simulink library "aerolibgravity2"  (R2020a)
settings: Solver=ode45  StartTime=0.0  StopTime=10.0  RelTol=1e-3
PostLoadFcn:
  | load_system('aerolibv1')
  | setsysloc('aerolibv1')
undefined symbols (not defined in the file or in its folder): aeroassertmsg, C, geoidgrid, ghCurrent, GM, latbp, lonbp, minYearCurrent, Newton, nMax10, nMax13, nMaxBetween, nMaxCurrent, R, Raphson, S, svCurrent, tabNMax10, tabNMax13, tabNMaxBetween
libraries: simulink x17, aerolibgravitysys x4
(part 3 of 4)

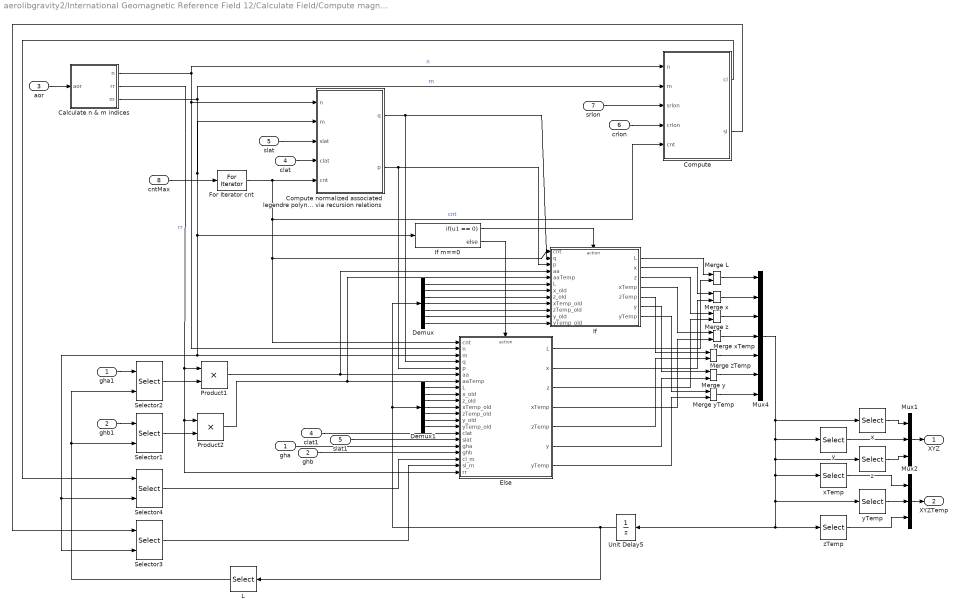
== system aerolibgravity2/International Geomagnetic Reference Field 12/Calculate Field/Compute magnetic vector in spherical coordinates/Compute magnetic vector in spherical coordinates ==
  gha : Inport  PortDimensions=(nMax13+1)*(nMax13+1)-1
  ghb : Inport  Port=2  PortDimensions=(nMax13+1)*(nMax13+1)-1
  aor : Inport  Port=3
  clat : Inport  Port=4
  slat : Inport  Port=5
  crlon : Inport  Port=6
  srlon : Inport  Port=7
  cntMax : Inport  Port=8
  Calculate n & m indices : Subsystem
  "Compute " : Subsystem
  Compute normalized associated legendre polynomials and derivatives via recursion relations : Subsystem
  Demux : Demux  Outputs=7
  Demux1 : Demux  Outputs=7
  Else : Subsystem
  For Iterator cnt : ForIterator  ResetStates=reset  IterationSource=external  IterationLimit=nPG
  If : Subsystem
  If m==0 : If  IfExpression=u1 == 0
  L : Selector  InputPortWidth=7  IndexOptions=Index vector (dialog)  Indices=1  OutputSizes=1
  Merge L : Merge  InitialOutput=0
  Merge x : Merge  InitialOutput=0
  Merge xTemp : Merge  InitialOutput=0
  Merge y : Merge  InitialOutput=0
  Merge yTemp : Merge  InitialOutput=0
  Merge z : Merge  InitialOutput=0
  Merge zTemp : Merge  InitialOutput=0
  Mux1 : Mux  Inputs=3
  Mux2 : Mux  Inputs=3
  Mux4 : Mux  Inputs=7
  Product1 : Product  SaturateOnIntegerOverflow=on  OutDataTypeStr=Inherit: Same as first input
  Product2 : Product  SaturateOnIntegerOverflow=on  OutDataTypeStr=Inherit: Same as first input
  Selector1 : Selector  InputPortWidth=(nMax13+1)*(nMax13+1)-1  IndexOptions=Index vector (port)  Indices=[1 3]  OutputSizes=1
  Selector2 : Selector  InputPortWidth=(nMax13+1)*(nMax13+1)-1  IndexOptions=Index vector (port)  Indices=[1 3]  OutputSizes=1
  Selector3 : Selector  IndexMode=Zero-based  InputPortWidth=nMax13+1  IndexOptions=Index vector (port)  Indices=[1 3]  OutputSizes=1
  Selector4 : Selector  IndexMode=Zero-based  InputPortWidth=nMax13+1  IndexOptions=Index vector (port)  Indices=[1 3]  OutputSizes=1
  Unit Delay5 : UnitDelay  InitialCondition=[1 0 0 0 0 0 0]  SampleTime=-1  HasFrameUpgradeWarning=on
  clat1 : InportShadow  Port=4
  gha1 : InportShadow  PortDimensions=(nMax13+1)*(nMax13+1)-1
  ghb1 : InportShadow  Port=2  PortDimensions=(nMax13+1)*(nMax13+1)-1
  slat1 : InportShadow  Port=5
  x : Selector  InputPortWidth=7  IndexOptions=Index vector (dialog)  Indices=2  OutputSizes=1
  xTemp : Selector  InputPortWidth=7  IndexOptions=Index vector (dialog)  Indices=4  OutputSizes=1
  y : Selector  InputPortWidth=7  IndexOptions=Index vector (dialog)  Indices=6  OutputSizes=1
  yTemp : Selector  InputPortWidth=7  IndexOptions=Index vector (dialog)  Indices=7  OutputSizes=1
  z : Selector  InputPortWidth=7  IndexOptions=Index vector (dialog)  Indices=3  OutputSizes=1
  zTemp : Selector  InputPortWidth=7  IndexOptions=Index vector (dialog)  Indices=5  OutputSizes=1
  XYZ : Outport  InitialOutput=[0 0 0]  VectorParamsAs1DForOutWhenUnconnected=off
  XYZTemp : Outport  Port=2  InitialOutput=[0 0 0]  VectorParamsAs1DForOutWhenUnconnected=off
  wires:
  yTemp/1 -> Mux2/2
  y/1 -> Mux1/2
  Demux1/7 -> Else/14(yTemp_old)
  Demux1/6 -> Else/13(y_old)
  Demux/7 -> If/12(yTemp_old)
  Demux/6 -> If/11(y_old)
  If/7(yTemp) -> Merge yTemp/1
  If/6(y) -> Merge y/1
  Else/7(yTemp) -> Merge yTemp/2
  cntMax/1 -> For Iterator cnt/1
  clat/1 -> Compute normalized associated legendre polynomials and derivatives via recursion relations/4(clat)
  slat/1 -> Compute normalized associated legendre polynomials and derivatives via recursion relations/3(slat)
  gha/1 -> Else/17(gha)
  ghb/1 -> Else/18(ghb)
  Mux2/1 -> XYZTemp/1
  Mux1/1 -> XYZ/1
  For Iterator cnt/1 -> Compute normalized associated legendre polynomials and derivatives via recursion relations/5(cnt), Else/1(cnt), If/1(cnt), "Compute "/5(cnt)  "cnt"
  If m==0/1 -> If/Action
  If m==0/2 -> Else/Action
  If/1("L ") -> Merge L/1
  If/2(x) -> Merge x/1
  If/3(z) -> Merge z/1
  If/4(xTemp) -> Merge xTemp/1
  If/5(zTemp) -> Merge zTemp/1
  Else/1("L ") -> Merge L/2
  Else/2(x) -> Merge x/2
  Else/3(z) -> Merge z/2
  Else/4(xTemp) -> Merge xTemp/2
  Else/5(zTemp) -> Merge zTemp/2
  Mux4/1 -> y/1, yTemp/1, Unit Delay5/1, zTemp/1, xTemp/1, z/1, x/1
  Else/6(y) -> Merge y/2
  Unit Delay5/1 -> Demux1/1, Demux/1, L/1
  Demux/1 -> If/6(L)
  Demux/3 -> If/8(z_old)
  Demux/2 -> If/7(x_old)
  Demux/4 -> If/9(xTemp_old)
  Demux/5 -> If/10(zTemp_old)
  Demux1/1 -> Else/8(L)
  Demux1/5 -> Else/12(zTemp_old)
  Demux1/4 -> Else/11(xTemp_old)
  Demux1/3 -> Else/10(z_old)
  Demux1/2 -> Else/9(x_old)
  xTemp/1 -> Mux2/1
  zTemp/1 -> Mux2/3
  x/1 -> Mux1/1
  z/1 -> Mux1/3
  Compute normalized associated legendre polynomials and derivatives via recursion relations/1(q) -> If/2(q), Else/4(q)
  Compute normalized associated legendre polynomials and derivatives via recursion relations/2(p) -> If/3(p), Else/5(p)
  Calculate n & m indices/2(rr) -> Product1/1, Else/21(rr), Product2/1  "rr"
  clat1/1 -> Else/15(clat)
  slat1/1 -> Else/16(slat)
  gha1/1 -> Selector2/1
  ghb1/1 -> Selector1/1
  L/1 -> Selector2/2, Selector1/2
  Selector2/1 -> Product1/2
  Product1/1 -> Else/6(aa), If/4(aa)
  Selector1/1 -> Product2/2
  Product2/1 -> Else/7(aaTemp), If/5(aaTemp)
  srlon/1 -> "Compute "/3(srlon)
  crlon/1 -> "Compute "/4(crlon)
  "Compute "/1(cl) -> Selector4/1
  Selector4/1 -> Else/19(cl_m)
  Selector3/1 -> Else/20(sl_m)
  "Compute "/2(sl) -> Selector3/1
  Calculate n & m indices/1(n) -> Else/2(n), Compute normalized associated legendre polynomials and derivatives via recursion relations/1(n), "Compute "/1(n)  "n"
  Calculate n & m indices/3(m) -> Compute normalized associated legendre polynomials and derivatives via recursion relations/2(m), Else/3(m), Selector4/2, Selector3/2, If m==0/1, "Compute "/2(m)  "m"
  aor/1 -> Calculate n & m indices/1(aor)
  Merge L/1 -> Mux4/1
  Merge x/1 -> Mux4/2
  Merge z/1 -> Mux4/3
  Merge y/1 -> Mux4/6
  Merge yTemp/1 -> Mux4/7
  Merge zTemp/1 -> Mux4/5
  Merge xTemp/1 -> Mux4/4

== system aerolibgravity2/International Geomagnetic Reference Field 12/Calculate Field/Convert from geodetic to spherical coordinates/calculate cd ==
  alt : Inport
  r : Inport  Port=2
  d : Inport  Port=3
  Product11 : Product  Inputs=*/  OutDataTypeStr=Inherit: Inherit via back propagation  SaturateOnIntegerOverflow=on
  Sum8 : Sum  Inputs=|++  OutDataTypeStr=Inherit: Inherit via back propagation  SaturateOnIntegerOverflow=on
  cd : Outport  VectorParamsAs1DForOutWhenUnconnected=off
  wires:
  Product11/1 -> cd/1
  d/1 -> Sum8/2
  alt/1 -> Sum8/1
  r/1 -> Product11/2
  Sum8/1 -> Product11/1

== system aerolibgravity2/International Geomagnetic Reference Field 12/Calculate Field/Convert from geodetic to spherical coordinates/calculate clat & slat ==
  sd : Inport
  srlat : Inport  Port=2
  crlat : Inport  Port=3
  cd : Inport  Port=4
  Product{1..4} (4 alike) : Product  OutDataTypeStr=Inherit: Inherit via back propagation  SaturateOnIntegerOverflow=on
  Sum1 : Sum  Inputs=|+-  OutDataTypeStr=Inherit: Inherit via back propagation  SaturateOnIntegerOverflow=on
  Sum2 : Sum  Inputs=|++  OutDataTypeStr=Inherit: Inherit via back propagation  SaturateOnIntegerOverflow=on
  "cd " : InportShadow  Port=4
  "crlat " : InportShadow  Port=3
  "sd " : InportShadow
  "srlat " : InportShadow  Port=2
  clat : Outport  VectorParamsAs1DForOutWhenUnconnected=off
  slat : Outport  Port=2  VectorParamsAs1DForOutWhenUnconnected=off
  wires:
  srlat/1 -> Product1/1
  cd/1 -> Product1/2
  sd/1 -> Product2/2
  crlat/1 -> Product2/1
  Product1/1 -> Sum1/1
  Product2/1 -> Sum1/2
  Sum1/1 -> slat/1
  "crlat "/1 -> Product3/1
  "cd "/1 -> Product3/2
  "srlat "/1 -> Product4/1
  "sd "/1 -> Product4/2
  Product4/1 -> Sum2/1
  Product3/1 -> Sum2/2
  Sum2/1 -> clat/1

== system aerolibgravity2/International Geomagnetic Reference Field 12/Calculate Field/Convert from geodetic to spherical coordinates/calculate d ==
  a2 : Inport
  b2 : Inport  Port=2
  srlat2 : Inport  Port=3
  crlat2 : Inport  Port=4
  Product10 : Product  OutDataTypeStr=Inherit: Inherit via back propagation  SaturateOnIntegerOverflow=on
  Product9 : Product  OutDataTypeStr=Inherit: Inherit via back propagation  SaturateOnIntegerOverflow=on
  Sum7 : Sum  Inputs=++|  OutDataTypeStr=Inherit: Inherit via back propagation  SaturateOnIntegerOverflow=on
  sqrt : Sqrt  OutDataTypeStr=Inherit: Inherit via back propagation  AlgorithmType=Newton-Raphson  SaturateOnIntegerOverflow=on
  c2 : Outport  VectorParamsAs1DForOutWhenUnconnected=off
  d : Outport  Port=2  VectorParamsAs1DForOutWhenUnconnected=off
  wires:
  sqrt/1 -> d/1  "d"
  srlat2/1 -> Product10/2
  b2/1 -> Product10/1
  a2/1 -> Product9/2
  crlat2/1 -> Product9/1
  Product10/1 -> Sum7/2
  Product9/1 -> Sum7/1
  Sum7/1 -> sqrt/1, c2/1

== system aerolibgravity2/International Geomagnetic Reference Field 12/Calculate Field/Convert from geodetic to spherical coordinates/calculate r2 ==
  alt : Inport
  a2 : Inport  Port=2
  b2 : Inport  Port=3
  srlat2 : Inport  Port=4
  crlat2 : Inport  Port=5
  c2 : Inport  Port=6
  d : Inport  Port=7
  Gain : Gain  Gain=2  OutDataTypeStr=Inherit: Inherit via back propagation  SaturateOnIntegerOverflow=on
  Product1 : Product  OutDataTypeStr=Inherit: Inherit via back propagation  SaturateOnIntegerOverflow=on
  Product2 : Product  OutDataTypeStr=Inherit: Inherit via back propagation  SaturateOnIntegerOverflow=on
  Product7 : Product  Inputs=*/  OutDataTypeStr=Inherit: Inherit via back propagation  SaturateOnIntegerOverflow=on
  Product8 : Product  OutDataTypeStr=Inherit: Inherit via back propagation  SaturateOnIntegerOverflow=on
  Sum1 : Sum  Inputs=|++  OutDataTypeStr=Inherit: Inherit via back propagation  SaturateOnIntegerOverflow=on
  Sum5 : Sum  Inputs=++|  OutDataTypeStr=Inherit: Inherit via back propagation  SaturateOnIntegerOverflow=on
  Sum6 : Sum  Inputs=|++  OutDataTypeStr=Inherit: Inherit via back propagation  SaturateOnIntegerOverflow=on
  a4 : Product  OutDataTypeStr=Inherit: Inherit via back propagation  SaturateOnIntegerOverflow=on
  b4 : Product  OutDataTypeStr=Inherit: Inherit via back propagation  SaturateOnIntegerOverflow=on
  sqrt : Sqrt  OutDataTypeStr=Inherit: Inherit via back propagation  AlgorithmType=Newton-Raphson  SaturateOnIntegerOverflow=on
  r : Outport  VectorParamsAs1DForOutWhenUnconnected=off
  wires:
  b2/1 -> b4/1, b4/2
  Sum5/1 -> Product1/1
  srlat2/1 -> Product8/2
  a2/1 -> a4/1, a4/2
  alt/1 -> Sum5/2, Product1/2
  d/1 -> Gain/1
  a4/1 -> Product2/2
  Product8/1 -> Sum6/2
  Sum6/1 -> Product7/1
  Product7/1 -> Sum1/2
  Gain/1 -> Sum5/1
  b4/1 -> Product8/1
  Product2/1 -> Sum6/1
  crlat2/1 -> Product2/1
  c2/1 -> Product7/2
  Sum1/1 -> sqrt/1
  Product1/1 -> Sum1/1
  sqrt/1 -> r/1

== system aerolibgravity2/International Geomagnetic Reference Field 12/Calculate Field/Convert from geodetic to spherical coordinates/calculate sd ==
  d : Inport
  a2 : Inport  Port=2
  b2 : Inport  Port=3
  r : Inport  Port=4
  crlat : Inport  Port=5
  srlat : Inport  Port=6
  Product1 : Product  OutDataTypeStr=Inherit: Inherit via back propagation  SaturateOnIntegerOverflow=on
  Product12 : Product  Inputs=*/**  OutDataTypeStr=Inherit: Inherit via back propagation  SaturateOnIntegerOverflow=on
  Sum1 : Sum  Inputs=|-+  OutDataTypeStr=Inherit: Inherit via back propagation  SaturateOnIntegerOverflow=on
  sd : Outport  VectorParamsAs1DForOutWhenUnconnected=off
  wires:
  Product1/1 -> Product12/2
  crlat/1 -> Product12/3
  srlat/1 -> Product12/4
  Product12/1 -> sd/1
  a2/1 -> Sum1/2
  b2/1 -> Sum1/1
  d/1 -> Product1/2
  r/1 -> Product1/1
  Sum1/1 -> Product12/1  "c2"

== system aerolibgravity2/International Geomagnetic Reference Field 12/Calculate Field/Get Cosine and Sine of Latitude and Longitude/300 ft from North & South poles ==
  "crlat " : Inport
  300 ft from pole : Constant  Value=89.999/180*pi
  >cos(89.999/180*pi) : Switch  Criteria=u2 > Threshold  Threshold=cos(89.999/180*pi)
  Trigonometric Function : Trigonometry  Operator=cos
  crlat : Outport  VectorParamsAs1DForOutWhenUnconnected=off
  wires:
  >cos(89.999/180*pi)/1 -> crlat/1
  "crlat "/1 -> >cos(89.999/180*pi)/2, >cos(89.999/180*pi)/1
  Trigonometric Function/1 -> >cos(89.999/180*pi)/3
  300 ft from pole/1 -> Trigonometric Function/1

== system aerolibgravity2/International Geomagnetic Reference Field 12/Calculate Field/Get Cosine and Sine of Latitude and Longitude/Angle Conversion ==
  in : Inport
  Unit Conversion : UnitConversion
  out : Outport  Unit=rad  VectorParamsAs1DForOutWhenUnconnected=off
  wires:
  Unit Conversion/1 -> out/1
  in/1 -> Unit Conversion/1

== system aerolibgravity2/International Geomagnetic Reference Field 12/Calculate H, F, DEC,& DIP/Else Action/Angle Conversion ==
  in : Inport  Unit=rad
  Unit Conversion : UnitConversion
  out : Outport  Unit=deg  VectorParamsAs1DForOutWhenUnconnected=off
  wires:
  in/1 -> Unit Conversion/1
  Unit Conversion/1 -> out/1

== system aerolibgravity2/International Geomagnetic Reference Field 12/Calculate H, F, DEC,& DIP/Else Action/Else Action ==
  H : Inport
  X : Inport  Port=2
  Y : Inport  Port=3
  Action Port : ActionPort
  Angle Conversion : Subsystem
  Gain : Gain  Gain=2
  Sum : Sum  Inputs=|++
  Switch : Switch  Threshold=0.0001
  Trigonometric Function : Trigonometry  Operator=atan2
  pi : Constant  Value=pi
  DEC : Outport  InitialOutput=0  VectorParamsAs1DForOutWhenUnconnected=off
  wires:
  Gain/1 -> Switch/1
  H/1 -> Sum/2
  X/1 -> Sum/1
  Y/1 -> Trigonometric Function/1
  Angle Conversion/1(out) -> DEC/1
  pi/1 -> Switch/3
  Sum/1 -> Trigonometric Function/2, Switch/2
  Switch/1 -> Angle Conversion/1(in)
  Trigonometric Function/1 -> Gain/1

== system aerolibgravity2/International Geomagnetic Reference Field 12/Calculate H, F, DEC,& DIP/Else Action/If Action ==
  Action Port : ActionPort
  NaN : Constant  Value=NaN
  DEC : Outport  Unit=deg  InitialOutput=0  VectorParamsAs1DForOutWhenUnconnected=off
  wires:
  NaN/1 -> DEC/1

== system aerolibgravity2/International Geomagnetic Reference Field 12/Calculate Secular Variation/Else Action/Angle Conversion ==
  in : Inport  Unit=rad
  Unit Conversion : UnitConversion
  out : Outport  Unit=deg  VectorParamsAs1DForOutWhenUnconnected=off
  wires:
  Unit Conversion/1 -> out/1
  in/1 -> Unit Conversion/1

== system aerolibgravity2/International Geomagnetic Reference Field 12/Calculate Secular Variation/Else Action/Else Action ==
  HTemp : Inport
  XTemp : Inport  Port=2
  YTemp : Inport  Port=3
  Action Port : ActionPort
  Angle Conversion : Subsystem
  Gain : Gain  Gain=2
  Sum : Sum  Inputs=|++
  Switch : Switch  Threshold=0.0001
  Trigonometric Function : Trigonometry  Operator=atan2
  pi : Constant  Value=pi
  DECTemp : Outport  Unit=deg  InitialOutput=0  VectorParamsAs1DForOutWhenUnconnected=off
  wires:
  Trigonometric Function/1 -> Gain/1
  Switch/1 -> Angle Conversion/1(in)
  Sum/1 -> Switch/2, Trigonometric Function/2
  pi/1 -> Switch/3
  Angle Conversion/1(out) -> DECTemp/1
  YTemp/1 -> Trigonometric Function/1
  XTemp/1 -> Sum/1
  HTemp/1 -> Sum/2
  Gain/1 -> Switch/1

== system aerolibgravity2/International Geomagnetic Reference Field 12/Calculate Secular Variation/Else Action/If Action ==
  Action Port : ActionPort
  NaN : Constant  Value=NaN
  DECTemp : Outport  Unit=deg  InitialOutput=0  VectorParamsAs1DForOutWhenUnconnected=off
  wires:
  NaN/1 -> DECTemp/1

== system aerolibgravity2/International Geomagnetic Reference Field 12/Extrapolate or Interpolate/Interpolate/1900-1990 ==
  dyear : Inport
  Action Port : ActionPort
  1 year/5 years : Bias  Bias=0.2
  1900-1990 Current : LookupNDDirect  InputsSelectThisObjectFromTable=Vector  Table=tabNMax10
  1900-1990 Next : LookupNDDirect  InputsSelectThisObjectFromTable=Vector  Table=tabNMax10
  Bias1 : Bias  Bias=1.0
  Constant : Constant  Value=nMax10
  Prelookup Current 1900-1990 : PreLookup  BreakpointsData=bpNMax10  IndexSearchMethod=Evenly spaced points  BeginIndexSearchUsingPreviousIndexResult=on  ExtrapMethod=Linear
  Product1 : Product  RndMeth=Zero
  Product2 : Product  RndMeth=Zero
  Sum1 : Sum  Inputs=-+|
  Sum2 : Sum  Inputs=++|
  Sum3 : Sum  Inputs=+|+
  gha : Outport  InitialOutput=zeros(195,1)  VectorParamsAs1DForOutWhenUnconnected=off
  ghb : Outport  Port=2  InitialOutput=zeros(195,1)  VectorParamsAs1DForOutWhenUnconnected=off
  nMax : Outport  Port=3  InitialOutput=nMax10  VectorParamsAs1DForOutWhenUnconnected=off
  wires:
  Bias1/1 -> 1900-1990 Next/1
  Prelookup Current 1900-1990/2 -> 1 year/5 years/1, Product2/1
  Prelookup Current 1900-1990/1 -> Bias1/1, 1900-1990 Current/1
  dyear/1 -> Prelookup Current 1900-1990/1
  1900-1990 Current/1 -> Sum1/1, Sum3/1, Sum2/1
  1900-1990 Next/1 -> Sum1/2
  1 year/5 years/1 -> Product1/2
  Sum1/1 -> Product2/2, Product1/1
  Product2/1 -> Sum2/2
  Sum2/1 -> gha/1
  Product1/1 -> Sum3/2
  Sum3/1 -> ghb/1
  Constant/1 -> nMax/1

== system aerolibgravity2/International Geomagnetic Reference Field 12/Extrapolate or Interpolate/Interpolate/1990-1995 ==
  dyear : Inport
  Action Port : ActionPort
  1 year/5 years : Bias  Bias=0.2
  1990-1995 Current : LookupNDDirect  InputsSelectThisObjectFromTable=Vector  Table=tabNMaxBetween
  1990-1995 Next : LookupNDDirect  InputsSelectThisObjectFromTable=Vector  Table=tabNMaxBetween
  Bias1 : Bias  Bias=1.0
  Constant : Constant  Value=nMaxBetween
  Prelookup Current 1990-1995 : PreLookup  BreakpointsData=bpNMaxBetween  IndexSearchMethod=Evenly spaced points  BeginIndexSearchUsingPreviousIndexResult=on  ExtrapMethod=Linear
  Product1 : Product  RndMeth=Zero
  Product2 : Product  RndMeth=Zero
  Sum1 : Sum  Inputs=-+|
  Sum2 : Sum  Inputs=++|
  Sum3 : Sum  Inputs=+|+
  gha : Outport  InitialOutput=zeros(195,1)  VectorParamsAs1DForOutWhenUnconnected=off
  ghb : Outport  Port=2  InitialOutput=zeros(195,1)  VectorParamsAs1DForOutWhenUnconnected=off
  nMax : Outport  Port=3  InitialOutput=nMaxBetween  VectorParamsAs1DForOutWhenUnconnected=off
  wires:
  Bias1/1 -> 1990-1995 Next/1
  Prelookup Current 1990-1995/2 -> 1 year/5 years/1, Product2/1
  Prelookup Current 1990-1995/1 -> Bias1/1, 1990-1995 Current/1
  dyear/1 -> Prelookup Current 1990-1995/1
  1990-1995 Current/1 -> Sum3/1, Sum2/1, Sum1/1
  1990-1995 Next/1 -> Sum1/2
  1 year/5 years/1 -> Product1/2
  Sum1/1 -> Product2/2, Product1/1
  Product2/1 -> Sum2/2
  Sum2/1 -> gha/1
  Product1/1 -> Sum3/2
  Sum3/1 -> ghb/1
  Constant/1 -> nMax/1

== system aerolibgravity2/International Geomagnetic Reference Field 12/Extrapolate or Interpolate/Interpolate/1995-2010 ==
  dyear : Inport
  Action Port : ActionPort
  1 year/5 years : Bias  Bias=0.2
  1995-2010 Current : LookupNDDirect  InputsSelectThisObjectFromTable=Vector  Table=tabNMax13
  1995-2010 Next : LookupNDDirect  InputsSelectThisObjectFromTable=Vector  Table=tabNMax13
  Bias1 : Bias  Bias=1.0
  Constant : Constant  Value=nMax13
  Prelookup Current 1995-2010 : PreLookup  BreakpointsData=bpNMax13  IndexSearchMethod=Evenly spaced points  BeginIndexSearchUsingPreviousIndexResult=on  ExtrapMethod=Linear
  Product1 : Product  RndMeth=Zero
  Product2 : Product  RndMeth=Zero
  Sum1 : Sum  Inputs=-+|
  Sum2 : Sum  Inputs=++|
  Sum3 : Sum  Inputs=+|+
  gha : Outport  InitialOutput=zeros(195,1)  VectorParamsAs1DForOutWhenUnconnected=off
  ghb : Outport  Port=2  InitialOutput=zeros(195,1)  VectorParamsAs1DForOutWhenUnconnected=off
  nMax : Outport  Port=3  InitialOutput=nMax13  VectorParamsAs1DForOutWhenUnconnected=off
  wires:
  Bias1/1 -> 1995-2010 Next/1
  Constant/1 -> nMax/1
  Sum3/1 -> ghb/1
  Product1/1 -> Sum3/2
  Sum2/1 -> gha/1
  Product2/1 -> Sum2/2
  Sum1/1 -> Product1/1, Product2/2
  1 year/5 years/1 -> Product1/2
  1995-2010 Next/1 -> Sum1/2
  1995-2010 Current/1 -> Sum1/1, Sum2/1, Sum3/1
  dyear/1 -> Prelookup Current 1995-2010/1
  Prelookup Current 1995-2010/1 -> Bias1/1, 1995-2010 Current/1
  Prelookup Current 1995-2010/2 -> 1 year/5 years/1, Product2/1

== system aerolibgravity2/International Geomagnetic Reference Field 12/Calculate Field/Compute magnetic vector in spherical coordinates/Compute magnetic vector in spherical coordinates/Calculate n & m indices ==
  aor : Inport
  If : If  NumInputs=2  IfExpression="u1 <=  u2"
  If Action Subsystem : Subsystem  TreatAsAtomicUnit=on
  If Action Subsystem1 : Subsystem  TreatAsAtomicUnit=on
  Merge1 : Merge
  Unit Delay1 : UnitDelay  SampleTime=-1  HasFrameUpgradeWarning=on
  Unit Delay2 : UnitDelay  SampleTime=-1  HasFrameUpgradeWarning=on
  n : Outport  VectorParamsAs1DForOutWhenUnconnected=off
  rr : Outport  Port=2  VectorParamsAs1DForOutWhenUnconnected=off
  m : Outport  Port=3  VectorParamsAs1DForOutWhenUnconnected=off
  wires:
  If/1 -> If Action Subsystem/Action
  Unit Delay2/1 -> If/1, If Action Subsystem/1("n ")
  Unit Delay1/1 -> If/2, If Action Subsystem1/1("m  ")
  If Action Subsystem/1(n) -> n/1, Unit Delay2/1  "n"
  Merge1/1 -> m/1, Unit Delay1/1  "m"
  aor/1 -> If Action Subsystem/2(aor)
  If/2 -> If Action Subsystem1/Action
  If Action Subsystem/3(m) -> Merge1/1  "m"
  If Action Subsystem1/1(m) -> Merge1/2
  If Action Subsystem/2(rr) -> rr/1

== system aerolibgravity2/International Geomagnetic Reference Field 12/Calculate Field/Compute magnetic vector in spherical coordinates/Compute magnetic vector in spherical coordinates/Compute  ==
  n : Inport
  m : Inport  Port=2
  srlon : Inport  Port=3
  crlon : Inport  Port=4
  cnt : Inport  Port=5
  Assignment1 : Assignment  IndexMode=Zero-based  DiagnosticForDimensions=Error  IndexOptions=Index vector (port)  Indices=1  OutputSizes=[1 1]
  Assignment2 : Assignment  IndexMode=Zero-based  DiagnosticForDimensions=Error  IndexOptions=Index vector (port)  Indices=1  OutputSizes=[1 1]
  Bus Creator1 : BusCreator  Inputs=4
  Else Subsystem : Subsystem
  If : If  IfExpression=u1 >=5
  If Subsystem : Subsystem
  Merge : Merge
  Merge1 : Merge
  Merge2 : Merge
  Unit Delay : UnitDelay  InitialCondition=zeros(nMax13+1,1)  SampleTime=-1  HasFrameUpgradeWarning=on
  Unit Delay1 : UnitDelay  InitialCondition=zeros(nMax13+1,1)  SampleTime=-1  HasFrameUpgradeWarning=on
  cl : Outport  VectorParamsAs1DForOutWhenUnconnected=off
  sl : Outport  Port=2  VectorParamsAs1DForOutWhenUnconnected=off
  wires:
  crlon/1 -> Else Subsystem/2(crlon)
  srlon/1 -> Else Subsystem/1(srlon)
  Merge1/1 -> Assignment2/2
  Merge2/1 -> Assignment2/3, Assignment1/3
  Merge/1 -> Assignment1/2
  Assignment1/1 -> Unit Delay/1, cl/1
  Else Subsystem/1(cl) -> Merge/2
  Else Subsystem/2(sl) -> Merge1/2
  Else Subsystem/3(idx0) -> Merge2/2
  If Subsystem/3(idx0) -> Merge2/1
  If Subsystem/1(cl) -> Merge/1
  If Subsystem/2(sl) -> Merge1/1
  If/2 -> Else Subsystem/Action
  Unit Delay/1 -> Bus Creator1/4, Assignment1/1  "cl_old"
  Unit Delay1/1 -> Bus Creator1/3, Assignment2/1  "sl_old"
  n/1 -> Bus Creator1/1
  If/1 -> If Subsystem/Action
  cnt/1 -> If/1
  Assignment2/1 -> Unit Delay1/1, sl/1
  Bus Creator1/1 -> If Subsystem/1(bus)
  m/1 -> Bus Creator1/2

== system aerolibgravity2/International Geomagnetic Reference Field 12/Calculate Field/Compute magnetic vector in spherical coordinates/Compute magnetic vector in spherical coordinates/Compute normalized associated legendre polynomials and derivatives via recursion relations ==
  n : Inport
  m : Inport  Port=2
  slat : Inport  Port=3
  clat : Inport  Port=4
  cnt : Inport  Port=5
  Bus Creator1 : BusCreator  Inputs=7
  Else Subsystem : Subsystem
  If : If  IfExpression=u1 >=5
  If Subsystem : Subsystem
  Merge : Merge
  Merge1 : Merge
  Unit Delay : UnitDelay  InitialCondition=zeros(nPG,1)  SampleTime=-1  HasFrameUpgradeWarning=on
  Unit Delay1 : UnitDelay  InitialCondition=zeros(nPG,1)  SampleTime=-1  HasFrameUpgradeWarning=on
  cnt1 : InportShadow  Port=5
  q : Outport  VectorParamsAs1DForOutWhenUnconnected=off
  p : Outport  Port=2  VectorParamsAs1DForOutWhenUnconnected=off
  wires:
  Else Subsystem/1(q) -> Merge1/2
  If Subsystem/1(q) -> Merge1/1
  Else Subsystem/2(p) -> Merge/2
  If Subsystem/2(p) -> Merge/1
  If/2 -> Else Subsystem/Action
  Unit Delay/1 -> Bus Creator1/7  "q_old"
  Unit Delay1/1 -> Bus Creator1/6  "p_old"
  cnt/1 -> Bus Creator1/5
  clat/1 -> Bus Creator1/4
  slat/1 -> Bus Creator1/3
  m/1 -> Bus Creator1/2
  n/1 -> Bus Creator1/1
  Bus Creator1/1 -> If Subsystem/2(bus), Else Subsystem/1(bus)
  Merge1/1 -> Unit Delay/1, q/1
  Merge/1 -> Unit Delay1/1, p/1
  cnt1/1 -> If Subsystem/1(cnt2), If/1
  If/1 -> If Subsystem/Action

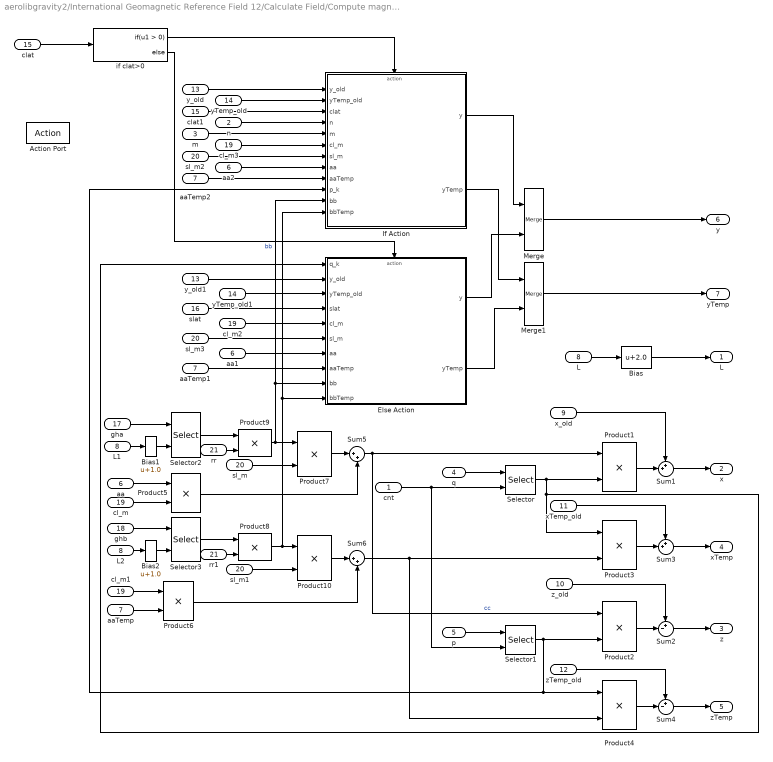
== system aerolibgravity2/International Geomagnetic Reference Field 12/Calculate Field/Compute magnetic vector in spherical coordinates/Compute magnetic vector in spherical coordinates/Else ==
  cnt : Inport
  n : Inport  Port=2
  m : Inport  Port=3
  q : Inport  Port=4
  p : Inport  Port=5
  aa : Inport  Port=6
  aaTemp : Inport  Port=7
  L : Inport  Port=8
  x_old : Inport  Port=9
  z_old : Inport  Port=10
  xTemp_old : Inport  Port=11
  zTemp_old : Inport  Port=12
  y_old : Inport  Port=13
  yTemp_old : Inport  Port=14
  clat : Inport  Port=15
  slat : Inport  Port=16
  gha : Inport  Port=17  PortDimensions=(nMax13+1)*(nMax13+1)-1
  ghb : Inport  Port=18  PortDimensions=(nMax13+1)*(nMax13+1)-1
  cl_m : Inport  Port=19
  sl_m : Inport  Port=20
  rr : Inport  Port=21
  Action Port : ActionPort
  Bias : Bias  Bias=2.0
  Bias1 : Bias  Bias=1.0
  Bias2 : Bias  Bias=1.0
  Else Action : Subsystem  TreatAsAtomicUnit=on
  If Action : Subsystem  TreatAsAtomicUnit=on
  L1 : InportShadow  Port=8
  L2 : InportShadow  Port=8
  Merge : Merge  InitialOutput=0
  Merge1 : Merge  InitialOutput=0
  Product{1..10} (10 alike) : Product  SaturateOnIntegerOverflow=on  OutDataTypeStr=Inherit: Same as first input
  Selector : Selector  InputPortWidth=nPG  IndexOptions=Index vector (port)  Indices=[1 3]  OutputSizes=1
  Selector1 : Selector  InputPortWidth=nPG  IndexOptions=Index vector (port)  Indices=[1 3]  OutputSizes=1
  Selector2 : Selector  InputPortWidth=(nMax13+1)*(nMax13+1)-1  IndexOptions=Index vector (port)  Indices=[1 3]  OutputSizes=1
  Selector3 : Selector  InputPortWidth=(nMax13+1)*(nMax13+1)-1  IndexOptions=Index vector (port)  Indices=[1 3]  OutputSizes=1
  Sum1 : Sum  Inputs=++|  SaturateOnIntegerOverflow=on
  Sum2 : Sum  Inputs=+-|  SaturateOnIntegerOverflow=on
  Sum3 : Sum  Inputs=++|  SaturateOnIntegerOverflow=on
  Sum4 : Sum  Inputs=+-|  SaturateOnIntegerOverflow=on
  Sum5 : Sum  Inputs=|++  SaturateOnIntegerOverflow=on
  Sum6 : Sum  Inputs=|++  SaturateOnIntegerOverflow=on
  aa1 : InportShadow  Port=6
  aa2 : InportShadow  Port=6
  aaTemp1 : InportShadow  Port=7
  aaTemp2 : InportShadow  Port=7
  cl_m1 : InportShadow  Port=19
  cl_m2 : InportShadow  Port=19
  cl_m3 : InportShadow  Port=19
  clat1 : InportShadow  Port=15
  if clat>0 : If
  rr1 : InportShadow  Port=21
  sl_m1 : InportShadow  Port=20
  sl_m2 : InportShadow  Port=20
  sl_m3 : InportShadow  Port=20
  yTemp_old1 : InportShadow  Port=14
  y_old1 : InportShadow  Port=13
  "L " : Outport  VectorParamsAs1DForOutWhenUnconnected=off
  x : Outport  Port=2  VectorParamsAs1DForOutWhenUnconnected=off
  z : Outport  Port=3  VectorParamsAs1DForOutWhenUnconnected=off
  xTemp : Outport  Port=4  VectorParamsAs1DForOutWhenUnconnected=off
  zTemp : Outport  Port=5  VectorParamsAs1DForOutWhenUnconnected=off
  y : Outport  Port=6  InitialOutput=0  VectorParamsAs1DForOutWhenUnconnected=off
  yTemp : Outport  Port=7  InitialOutput=0  VectorParamsAs1DForOutWhenUnconnected=off
  wires:
  yTemp_old/1 -> If Action/2(yTemp_old)
  y_old/1 -> If Action/1(y_old)
  yTemp_old1/1 -> Else Action/3(yTemp_old)
  y_old1/1 -> Else Action/2(y_old)
  Bias2/1 -> Selector3/2
  Bias1/1 -> Selector2/2
  if clat>0/2 -> Else Action/Action
  If Action/2(yTemp) -> Merge1/1
  If Action/1(y) -> Merge/1
  Else Action/2(yTemp) -> Merge1/2
  Else Action/1(y) -> Merge/2
  if clat>0/1 -> If Action/Action
  Merge1/1 -> yTemp/1
  Merge/1 -> y/1
  L/1 -> Bias/1
  Bias/1 -> "L "/1
  clat/1 -> if clat>0/1
  Sum1/1 -> x/1
  cnt/1 -> Selector1/2, Selector/2
  Product1/1 -> Sum1/2
  q/1 -> Selector/1
  Sum2/1 -> z/1
  Product2/1 -> Sum2/2
  Sum5/1 -> Product1/1, Product2/1  "cc"
  Sum3/1 -> xTemp/1
  Product3/1 -> Sum3/2
  Sum4/1 -> zTemp/1
  Product4/1 -> Sum4/2
  Sum6/1 -> Product3/2, Product4/2
  Selector/1 -> Product1/2, Product3/1, Else Action/1(q_k)
  Selector1/1 -> Product2/2, If Action/10(p_k), Product4/1
  p/1 -> Selector1/1
  x_old/1 -> Sum1/1
  z_old/1 -> Sum2/1
  xTemp_old/1 -> Sum3/1
  zTemp_old/1 -> Sum4/1
  aa/1 -> Product5/1
  cl_m/1 -> Product5/2
  aaTemp/1 -> Product6/2
  cl_m1/1 -> Product6/1
  gha/1 -> Selector2/1
  Selector2/1 -> Product9/1
  rr/1 -> Product9/2
  sl_m/1 -> Product7/2
  Product5/1 -> Sum5/2
  Product7/1 -> Sum5/1
  Product6/1 -> Sum6/2
  Product10/1 -> Sum6/1
  sl_m1/1 -> Product10/2
  rr1/1 -> Product8/2
  Selector3/1 -> Product8/1
  ghb/1 -> Selector3/1
  L1/1 -> Bias1/1
  L2/1 -> Bias2/1
  Product9/1 -> If Action/11(bb), Else Action/9(bb), Product7/1  "bb"
  Product8/1 -> Product10/1, If Action/12(bbTemp), Else Action/10(bbTemp)
  aa1/1 -> Else Action/7(aa)
  aa2/1 -> If Action/8(aa)
  aaTemp1/1 -> Else Action/8(aaTemp)
  aaTemp2/1 -> If Action/9(aaTemp)
  cl_m2/1 -> Else Action/5(cl_m)
  cl_m3/1 -> If Action/6(cl_m)
  sl_m2/1 -> If Action/7(sl_m)
  sl_m3/1 -> Else Action/6(sl_m)
  clat1/1 -> If Action/3(clat)
  slat/1 -> Else Action/4(slat)
  m/1 -> If Action/5(m)
  n/1 -> If Action/4(n)

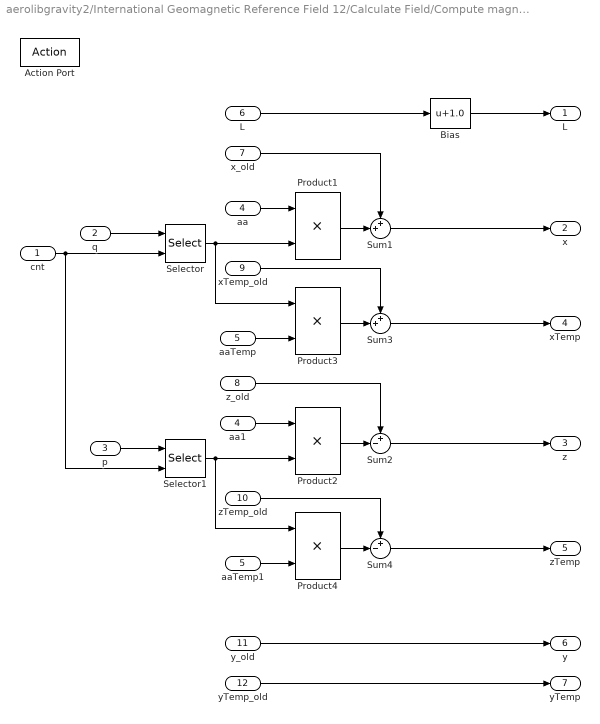
== system aerolibgravity2/International Geomagnetic Reference Field 12/Calculate Field/Compute magnetic vector in spherical coordinates/Compute magnetic vector in spherical coordinates/If ==
  cnt : Inport
  q : Inport  Port=2
  p : Inport  Port=3
  aa : Inport  Port=4
  aaTemp : Inport  Port=5
  L : Inport  Port=6
  x_old : Inport  Port=7
  z_old : Inport  Port=8
  xTemp_old : Inport  Port=9
  zTemp_old : Inport  Port=10
  y_old : Inport  Port=11
  yTemp_old : Inport  Port=12
  Action Port : ActionPort
  Bias : Bias  Bias=1.0
  Product{1..4} (4 alike) : Product  SaturateOnIntegerOverflow=on  OutDataTypeStr=Inherit: Same as first input
  Selector : Selector  InputPortWidth=nPG  IndexOptions=Index vector (port)  Indices=[1 3]  OutputSizes=1
  Selector1 : Selector  InputPortWidth=nPG  IndexOptions=Index vector (port)  Indices=[1 3]  OutputSizes=1
  Sum1 : Sum  Inputs=++|  SaturateOnIntegerOverflow=on
  Sum2 : Sum  Inputs=+-|  SaturateOnIntegerOverflow=on
  Sum3 : Sum  Inputs=++|  SaturateOnIntegerOverflow=on
  Sum4 : Sum  Inputs=+-|  SaturateOnIntegerOverflow=on
  aa1 : InportShadow  Port=4
  aaTemp1 : InportShadow  Port=5
  "L " : Outport  VectorParamsAs1DForOutWhenUnconnected=off
  x : Outport  Port=2  VectorParamsAs1DForOutWhenUnconnected=off
  z : Outport  Port=3  VectorParamsAs1DForOutWhenUnconnected=off
  xTemp : Outport  Port=4  VectorParamsAs1DForOutWhenUnconnected=off
  zTemp : Outport  Port=5  VectorParamsAs1DForOutWhenUnconnected=off
  y : Outport  Port=6  InitialOutput=0  VectorParamsAs1DForOutWhenUnconnected=off
  yTemp : Outport  Port=7  InitialOutput=0  VectorParamsAs1DForOutWhenUnconnected=off
  wires:
  yTemp_old/1 -> yTemp/1
  y_old/1 -> y/1
  Sum1/1 -> x/1
  cnt/1 -> Selector/2, Selector1/2
  Product1/1 -> Sum1/2
  q/1 -> Selector/1
  Sum2/1 -> z/1
  Product2/1 -> Sum2/2
  L/1 -> Bias/1
  Bias/1 -> "L "/1
  aa/1 -> Product1/1
  aa1/1 -> Product2/1
  Sum3/1 -> xTemp/1
  Product3/1 -> Sum3/2
  Sum4/1 -> zTemp/1
  Product4/1 -> Sum4/2
  aaTemp/1 -> Product3/2
  aaTemp1/1 -> Product4/2
  Selector/1 -> Product1/2, Product3/1
  Selector1/1 -> Product2/2, Product4/1
  p/1 -> Selector1/1
  x_old/1 -> Sum1/1
  z_old/1 -> Sum2/1
  xTemp_old/1 -> Sum3/1
  zTemp_old/1 -> Sum4/1

== system aerolibgravity2/International Geomagnetic Reference Field 12/Calculate H, F, DEC,& DIP/Else Action/Else Action/Angle Conversion ==
  in : Inport  Unit=rad
  Unit Conversion : UnitConversion
  out : Outport  Unit=deg  VectorParamsAs1DForOutWhenUnconnected=off
  wires:
  in/1 -> Unit Conversion/1
  Unit Conversion/1 -> out/1

== system aerolibgravity2/International Geomagnetic Reference Field 12/Calculate Secular Variation/Else Action/Else Action/Angle Conversion ==
  in : Inport  Unit=rad
  Unit Conversion : UnitConversion
  out : Outport  Unit=deg  VectorParamsAs1DForOutWhenUnconnected=off
  wires:
  Unit Conversion/1 -> out/1
  in/1 -> Unit Conversion/1

== system aerolibgravity2/International Geomagnetic Reference Field 12/Calculate Field/Compute magnetic vector in spherical coordinates/Compute magnetic vector in spherical coordinates/Calculate n & m indices/If Action Subsystem ==
  "n " : Inport
  aor : Inport  Port=2
  Action Port : ActionPort
  Constant2 : Constant  Value=0.0  OutDataTypeStr=Inherit: Inherit via back propagation
  Math Function : Math  Operator=pow  SignedPower=on  SaturateOnIntegerOverflow=on
  n+1 : Bias  Bias=1.0
  n+2 : Bias  Bias=2.0
  n : Outport  InitialOutput=0  VectorParamsAs1DForOutWhenUnconnected=off
  rr : Outport  Port=2  InitialOutput=0  VectorParamsAs1DForOutWhenUnconnected=off
  m : Outport  Port=3  InitialOutput=0  VectorParamsAs1DForOutWhenUnconnected=off
  wires:
  "n "/1 -> n+1/1
  Constant2/1 -> m/1
  n+1/1 -> n/1, n+2/1
  aor/1 -> Math Function/1
  n+2/1 -> Math Function/2
  Math Function/1 -> rr/1

== system aerolibgravity2/International Geomagnetic Reference Field 12/Calculate Field/Compute magnetic vector in spherical coordinates/Compute magnetic vector in spherical coordinates/Calculate n & m indices/If Action Subsystem1 ==
  "m  " : Inport
  Action Port : ActionPort
  m+1 : Bias  Bias=1.0
  m : Outport  VectorParamsAs1DForOutWhenUnconnected=off
  wires:
  m+1/1 -> m/1
  "m  "/1 -> m+1/1

== system aerolibgravity2/International Geomagnetic Reference Field 12/Calculate Field/Compute magnetic vector in spherical coordinates/Compute magnetic vector in spherical coordinates/Compute /Else Subsystem ==
  srlon : Inport
  crlon : Inport  Port=2
  Action Port : ActionPort
  Constant3 : Constant  OutDataTypeStr=Inherit: Inherit via back propagation
  cl : Outport  InitialOutput=0  VectorParamsAs1DForOutWhenUnconnected=off
  sl : Outport  Port=2  InitialOutput=0  VectorParamsAs1DForOutWhenUnconnected=off
  idx0 : Outport  Port=3  InitialOutput=1  VectorParamsAs1DForOutWhenUnconnected=off
  wires:
  Constant3/1 -> idx0/1
  srlon/1 -> sl/1
  crlon/1 -> cl/1

== system aerolibgravity2/International Geomagnetic Reference Field 12/Calculate Field/Compute magnetic vector in spherical coordinates/Compute magnetic vector in spherical coordinates/Compute /If Subsystem ==
  bus : Inport
  Action Port : ActionPort
  Bus Selector3 : BusSelector  OutputSignals=sl_old,cl_old,m
  Bus Selector5 : BusSelector  OutputSignals=n,m
  If Action Subsystem : Subsystem  TreatAsAtomicUnit=on
  if n == m : If  NumInputs=2  IfExpression=u1 == u2  ShowElse=off
  cl : Outport  VectorParamsAs1DForOutWhenUnconnected=off
  sl : Outport  Port=2  VectorParamsAs1DForOutWhenUnconnected=off
  idx0 : Outport  Port=3  VectorParamsAs1DForOutWhenUnconnected=off
  wires:
  If Action Subsystem/3(Idx0) -> idx0/1
  Bus Selector5/2 -> if n == m/2  "<m>"
  Bus Selector5/1 -> if n == m/1  "<n>"
  if n == m/1 -> If Action Subsystem/Action
  If Action Subsystem/2(cl) -> cl/1
  If Action Subsystem/1(sl) -> sl/1
  bus/1 -> Bus Selector3/1, Bus Selector5/1
  Bus Selector3/1 -> If Action Subsystem/1(sl_old)  "<sl_old>"
  Bus Selector3/2 -> If Action Subsystem/2(cl_old)  "<cl_old>"
  Bus Selector3/3 -> If Action Subsystem/3(m)  "<m>"

== system aerolibgravity2/International Geomagnetic Reference Field 12/Calculate Field/Compute magnetic vector in spherical coordinates/Compute magnetic vector in spherical coordinates/Compute normalized associated legendre polynomials and derivatives via recursion relations/Else Subsystem ==
  bus : Inport
  Action Port : ActionPort
  Assignment2 : Assignment  DiagnosticForDimensions=Error  IndexOptions=Index vector (dialog)  Indices=1:4  OutputSizes=[1 1]
  Assignment3 : Assignment  DiagnosticForDimensions=Error  IndexOptions=Index vector (dialog)  Indices=1:4  OutputSizes=[1 1]
  Bus Selector2 : BusSelector  OutputSignals=p_old
  Bus Selector4 : BusSelector  OutputSignals=q_old
  Gain1 : Gain
  Gain2 : Gain
  p(1:4) : Subsystem
  q(1:4) : Subsystem
  q : Outport  VectorParamsAs1DForOutWhenUnconnected=off
  p : Outport  Port=2  VectorParamsAs1DForOutWhenUnconnected=off
  wires:
  Gain2/1 -> q/1
  Gain1/1 -> p/1
  Assignment3/1 -> Gain1/1
  p(1:4)/1(p(1:4)) -> Assignment3/2
  Assignment2/1 -> Gain2/1
  q(1:4)/1(q(1:4)) -> Assignment2/2
  bus/1 -> Bus Selector2/1, Bus Selector4/1, q(1:4)/1(bus), p(1:4)/1(bus)
  Bus Selector4/1 -> Assignment2/1  "<q_old>"
  Bus Selector2/1 -> Assignment3/1  "<p_old>"

== system aerolibgravity2/International Geomagnetic Reference Field 12/Calculate Field/Compute magnetic vector in spherical coordinates/Compute magnetic vector in spherical coordinates/Compute normalized associated legendre polynomials and derivatives via recursion relations/If Subsystem ==
  cnt2 : Inport
  bus : Inport  Port=2
  Action Port : ActionPort
  Assignment : Assignment  DiagnosticForDimensions=Error  IndexOptions=Index vector (port)  Indices=1  OutputSizes=1
  Assignment1 : Assignment  DiagnosticForDimensions=Error  IndexOptions=Index vector (port)  Indices=1  OutputSizes=[1 1]
  Assignment2 : Assignment  DiagnosticForDimensions=Error  IndexOptions=Index vector (dialog)  Indices=1:4  OutputSizes=[1 1]
  Assignment3 : Assignment  DiagnosticForDimensions=Error  IndexOptions=Index vector (dialog)  Indices=1:4  OutputSizes=[1 1]
  Bus Selector1 : BusSelector  OutputSignals=p_old,q_old,clat,slat,n,m,cnt
  Bus Selector2 : BusSelector  OutputSignals=p_old
  Bus Selector3 : BusSelector  OutputSignals=p_old,q_old,clat,slat,n,m,cnt
  Bus Selector4 : BusSelector  OutputSignals=q_old
  Bus Selector5 : BusSelector  OutputSignals=n,m
  Gain : Gain
  Gain1 : Gain
  If Action Subsystem : Subsystem  TreatAsAtomicUnit=on
  If Action Subsystem2 : Subsystem  TreatAsAtomicUnit=on
  Merge : Merge  InitialOutput=0
  Merge1 : Merge  InitialOutput=0
  cnt1 : InportShadow
  if n == m : If  NumInputs=2  IfExpression=u1 == u2
  p(1:4) : Subsystem
  q(1:4) : Subsystem
  q : Outport  VectorParamsAs1DForOutWhenUnconnected=off
  p : Outport  Port=2  VectorParamsAs1DForOutWhenUnconnected=off
  wires:
  Gain1/1 -> p/1
  Gain/1 -> q/1
  Bus Selector2/1 -> Assignment3/1  "<p_old>"
  Bus Selector4/1 -> Assignment2/1  "<q_old>"
  cnt2/1 -> Assignment/3
  bus/1 -> Bus Selector5/1, Bus Selector3/1, Bus Selector4/1, Bus Selector2/1, p(1:4)/1(bus), q(1:4)/1(bus), Bus Selector1/1
  if n == m/2 -> If Action Subsystem2/Action
  Merge1/1 -> Assignment/2
  Merge/1 -> Assignment1/2
  If Action Subsystem/2(q) -> Merge1/1
  If Action Subsystem/1(p) -> Merge/1
  If Action Subsystem2/2(q) -> Merge1/2
  If Action Subsystem2/1(p) -> Merge/2
  cnt1/1 -> Assignment1/3
  Assignment1/1 -> Gain1/1
  Assignment/1 -> Gain/1
  if n == m/1 -> If Action Subsystem/Action
  Bus Selector5/1 -> if n == m/1  "<n>"
  Bus Selector5/2 -> if n == m/2  "<m>"
  q(1:4)/1(q(1:4)) -> Assignment2/2
  Assignment2/1 -> Assignment/1
  p(1:4)/1(p(1:4)) -> Assignment3/2
  Assignment3/1 -> Assignment1/1
  Bus Selector3/1 -> If Action Subsystem/1(p_old)  "<p_old>"
  Bus Selector3/2 -> If Action Subsystem/2(q_old)  "<q_old>"
  Bus Selector3/3 -> If Action Subsystem/3(clat)  "<clat>"
  Bus Selector3/4 -> If Action Subsystem/4(slat)  "<slat>"
  Bus Selector3/5 -> If Action Subsystem/5(n)  "<n>"
  Bus Selector3/6 -> If Action Subsystem/6(m)  "<m>"
  Bus Selector3/7 -> If Action Subsystem/7(cnt)  "<cnt>"
  Bus Selector1/1 -> If Action Subsystem2/1(p_old)  "<p_old>"
  Bus Selector1/2 -> If Action Subsystem2/2(q_old)  "<q_old>"
  Bus Selector1/3 -> If Action Subsystem2/3(clat)  "<clat>"
  Bus Selector1/4 -> If Action Subsystem2/4(slat)  "<slat>"
  Bus Selector1/5 -> If Action Subsystem2/5(n)  "<n>"
  Bus Selector1/6 -> If Action Subsystem2/6(m)  "<m>"
  Bus Selector1/7 -> If Action Subsystem2/7(cnt)  "<cnt>"

== system aerolibgravity2/International Geomagnetic Reference Field 12/Calculate Field/Compute magnetic vector in spherical coordinates/Compute magnetic vector in spherical coordinates/Else/Else Action ==
  q_k : Inport
  y_old : Inport  Port=2
  yTemp_old : Inport  Port=3
  slat : Inport  Port=4
  cl_m : Inport  Port=5
  sl_m : Inport  Port=6
  aa : Inport  Port=7
  aaTemp : Inport  Port=8
  bb : Inport  Port=9
  bbTemp : Inport  Port=10
  Action Port : ActionPort
  Product{1..7} (7 alike) : Product  SaturateOnIntegerOverflow=on  OutDataTypeStr=Inherit: Same as first input
  Sum : Sum  Inputs=++|  SaturateOnIntegerOverflow=on
  Sum1 : Sum  Inputs=++|  SaturateOnIntegerOverflow=on
  Sum2 : Sum  Inputs=+-|  SaturateOnIntegerOverflow=on
  Sum3 : Sum  Inputs=|+-  SaturateOnIntegerOverflow=on
  cl_m1 : InportShadow  Port=5
  sl_m1 : InportShadow  Port=6
  y : Outport  InitialOutput=0  VectorParamsAs1DForOutWhenUnconnected=off
  yTemp : Outport  Port=2  InitialOutput=0  VectorParamsAs1DForOutWhenUnconnected=off
  wires:
  Sum1/1 -> yTemp/1
  yTemp_old/1 -> Sum1/1
  y_old/1 -> Sum/1
  Sum/1 -> y/1
  q_k/1 -> Product3/1
  slat/1 -> Product3/2
  Product6/1 -> Sum/2
  Product1/1 -> Sum1/2
  Product3/1 -> Product1/1, Product6/2
  Sum2/1 -> Product6/1
  Sum3/1 -> Product1/2
  bbTemp/1 -> Product4/2
  aaTemp/1 -> Product2/2
  sl_m/1 -> Product2/1
  cl_m/1 -> Product4/1
  Product2/1 -> Sum3/1
  Product4/1 -> Sum3/2
  Product5/1 -> Sum2/1
  Product7/1 -> Sum2/2
  aa/1 -> Product5/2
  bb/1 -> Product7/2
  cl_m1/1 -> Product7/1
  sl_m1/1 -> Product5/1

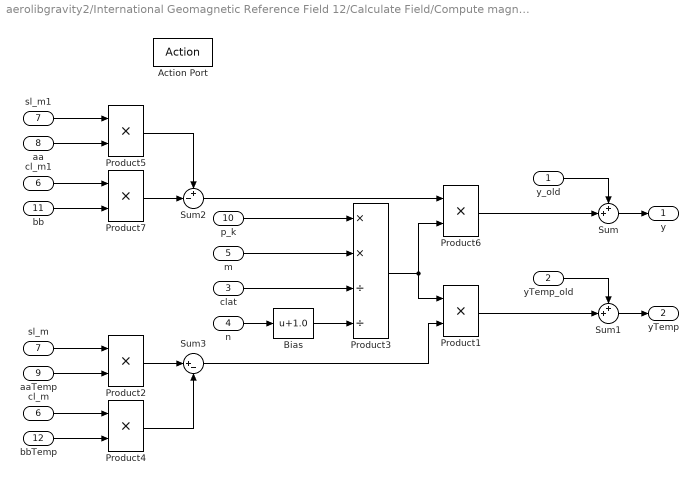
== system aerolibgravity2/International Geomagnetic Reference Field 12/Calculate Field/Compute magnetic vector in spherical coordinates/Compute magnetic vector in spherical coordinates/Else/If Action ==
  y_old : Inport
  yTemp_old : Inport  Port=2
  clat : Inport  Port=3
  n : Inport  Port=4
  m : Inport  Port=5
  cl_m : Inport  Port=6
  sl_m : Inport  Port=7
  aa : Inport  Port=8
  aaTemp : Inport  Port=9
  p_k : Inport  Port=10
  bb : Inport  Port=11
  bbTemp : Inport  Port=12
  Action Port : ActionPort
  Bias : Bias  Bias=1.0
  Product{1..2,4..7} (6 alike) : Product  SaturateOnIntegerOverflow=on  OutDataTypeStr=Inherit: Same as first input
  Product3 : Product  Inputs=**//  SaturateOnIntegerOverflow=on  OutDataTypeStr=Inherit: Same as first input
  Sum : Sum  Inputs=++|  SaturateOnIntegerOverflow=on
  Sum1 : Sum  Inputs=++|  SaturateOnIntegerOverflow=on
  Sum2 : Sum  Inputs=+-|  SaturateOnIntegerOverflow=on
  Sum3 : Sum  Inputs=|+-  SaturateOnIntegerOverflow=on
  cl_m1 : InportShadow  Port=6
  sl_m1 : InportShadow  Port=7
  y : Outport  VectorParamsAs1DForOutWhenUnconnected=off
  yTemp : Outport  Port=2  VectorParamsAs1DForOutWhenUnconnected=off
  wires:
  Sum1/1 -> yTemp/1
  yTemp_old/1 -> Sum1/1
  y_old/1 -> Sum/1
  Sum/1 -> y/1
  n/1 -> Bias/1
  p_k/1 -> Product3/1
  m/1 -> Product3/2
  clat/1 -> Product3/3
  Bias/1 -> Product3/4
  Product6/1 -> Sum/2
  Product1/1 -> Sum1/2
  Product3/1 -> Product6/2, Product1/1
  Sum2/1 -> Product6/1
  Sum3/1 -> Product1/2
  bbTemp/1 -> Product4/2
  aaTemp/1 -> Product2/2
  sl_m/1 -> Product2/1
  cl_m/1 -> Product4/1
  Product2/1 -> Sum3/1
  Product4/1 -> Sum3/2
  Product5/1 -> Sum2/1
  Product7/1 -> Sum2/2
  aa/1 -> Product5/2
  bb/1 -> Product7/2
  cl_m1/1 -> Product7/1
  sl_m1/1 -> Product5/1

== system aerolibgravity2/International Geomagnetic Reference Field 12/Calculate Field/Compute magnetic vector in spherical coordinates/Compute magnetic vector in spherical coordinates/Compute /If Subsystem/If Action Subsystem ==
  sl_old : Inport
  cl_old : Inport  Port=2
  m : Inport  Port=3
  Action Port : ActionPort  PropagateVarSize=During execution
  Bias : Bias  Bias=-1.0
  Constant2 : Constant  OutDataTypeStr=Inherit: Inherit via back propagation
  Demux : Demux  Outputs=2
  Demux1 : Demux  Outputs=2
  Gain : Gain
  Mux : Mux  Inputs=2
  Product : Product  Inputs=1  SaturateOnIntegerOverflow=on  OutDataTypeStr=Inherit: Same as first input
  Product1 : Product  SaturateOnIntegerOverflow=on  OutDataTypeStr=Inherit: Same as first input
  Product2 : Product  Inputs=1  SaturateOnIntegerOverflow=on  OutDataTypeStr=Inherit: Same as first input
  Product3 : Product  SaturateOnIntegerOverflow=on  OutDataTypeStr=Inherit: Same as first input
  Selector : Selector  IndexMode=Zero-based  InputPortWidth=nMax13+1  IndexOptions=Index vector (port)  Indices=[1 3]  OutputSizes=1
  Selector1 : Selector  IndexMode=Zero-based  InputPortWidth=nMax13+1  IndexOptions=Index vector (port)  Indices=1  OutputSizes=1
  Sum : Sum  Inputs=|-+  SaturateOnIntegerOverflow=on
  Sum1 : Sum  Inputs=|++  SaturateOnIntegerOverflow=on
  "m " : InportShadow  Port=3
  sl : Outport  InitialOutput=0  VectorParamsAs1DForOutWhenUnconnected=off
  cl : Outport  Port=2  InitialOutput=0  VectorParamsAs1DForOutWhenUnconnected=off
  Idx0 : Outport  Port=3  InitialOutput=1  VectorParamsAs1DForOutWhenUnconnected=off
  wires:
  Gain/1 -> Idx0/1
  "m "/1 -> Gain/1
  sl_old/1 -> Selector/1
  cl_old/1 -> Selector1/1
  Selector1/1 -> Product/1, Demux1/1
  Sum/1 -> cl/1
  Product/1 -> Sum/2
  Sum1/1 -> sl/1
  m/1 -> Bias/1
  Bias/1 -> Mux/1
  Constant2/1 -> Mux/2
  Mux/1 -> Selector/2, Selector1/2
  Selector/1 -> Product2/1, Demux/1
  Product2/1 -> Sum/1
  Product1/1 -> Sum1/1
  Product3/1 -> Sum1/2
  Demux/1 -> Product3/1
  Demux1/2 -> Product3/2
  Demux1/1 -> Product1/2
  Demux/2 -> Product1/1

== system aerolibgravity2/International Geomagnetic Reference Field 12/Calculate Field/Compute magnetic vector in spherical coordinates/Compute magnetic vector in spherical coordinates/Compute normalized associated legendre polynomials and derivatives via recursion relations/Else Subsystem/p(1:4) ==
  bus : Inport
  Bus Selector2 : BusSelector  OutputSignals=slat,clat,slat,slat,clat
  Constant : Constant  Value=3
  Constant1 : Constant  Value=1.5
  Gain : Gain  Gain=4.5
  Gain1 : Gain  Gain=2
  Gain2 : Gain  Gain=2
  Product3 : Product  Inputs=4  SaturateOnIntegerOverflow=on  OutDataTypeStr=Inherit: Same as first input
  Product4 : Product  SaturateOnIntegerOverflow=on  OutDataTypeStr=Inherit: Same as first input
  Sqrt : Sqrt  SaturateOnIntegerOverflow=on
  Sum2 : Sum  Inputs=-+|  SaturateOnIntegerOverflow=on
  Vector Concatenate : Concatenate  NumInputs=4
  p(1:4) : Outport  VectorParamsAs1DForOutWhenUnconnected=off
  wires:
  Bus Selector2/3 -> Product4/1, Product4/2  "<slat>"
  Bus Selector2/4 -> Product3/1  "<slat>"
  Bus Selector2/2 -> Gain2/1  "<clat>"
  Bus Selector2/1 -> Gain1/1  "<slat>"
  Constant1/1 -> Sum2/1
  Gain2/1 -> Vector Concatenate/2
  Gain1/1 -> Vector Concatenate/1
  Product4/1 -> Gain/1
  Sum2/1 -> Vector Concatenate/3
  Gain/1 -> Sum2/2
  Bus Selector2/5 -> Product3/2  "<clat>"
  Sqrt/1 -> Product3/4
  Product3/1 -> Vector Concatenate/4
  Constant/1 -> Product3/3, Sqrt/1
  bus/1 -> Bus Selector2/1
  Vector Concatenate/1 -> p(1:4)/1

== system aerolibgravity2/International Geomagnetic Reference Field 12/Calculate Field/Compute magnetic vector in spherical coordinates/Compute magnetic vector in spherical coordinates/Compute normalized associated legendre polynomials and derivatives via recursion relations/Else Subsystem/q(1:4) ==
  bus : Inport
  Bus Selector2 : BusSelector  OutputSignals=clat,slat,slat,clat,slat,clat
  Constant : Constant  Value=3
  Gain : Gain  Gain=3
  Product{1..4} (4 alike) : Product  SaturateOnIntegerOverflow=on  OutDataTypeStr=Inherit: Same as first input
  Sqrt : Sqrt  SaturateOnIntegerOverflow=on
  Sum1 : Sum  Inputs=+-|  SaturateOnIntegerOverflow=on
  Unary Minus : UnaryMinus
  Unary Minus1 : UnaryMinus
  Vector Concatenate : Concatenate  NumInputs=4
  q(1:4) : Outport  VectorParamsAs1DForOutWhenUnconnected=off
  wires:
  Bus Selector2/2 -> Vector Concatenate/2  "<slat>"
  Bus Selector2/1 -> Unary Minus/1  "<clat>"
  Vector Concatenate/1 -> q(1:4)/1
  bus/1 -> Bus Selector2/1
  Constant/1 -> Sqrt/1
  Product3/1 -> Vector Concatenate/4
  Sqrt/1 -> Product3/2
  Sum1/1 -> Product3/1
  Product1/1 -> Sum1/1
  Product2/1 -> Sum1/2
  Bus Selector2/6 -> Product2/2, Product2/1  "<clat>"
  Bus Selector2/5 -> Product1/1, Product1/2  "<slat>"
  Gain/1 -> Unary Minus1/1
  Unary Minus1/1 -> Vector Concatenate/3
  Product4/1 -> Gain/1
  Bus Selector2/4 -> Product4/2  "<clat>"
  Bus Selector2/3 -> Product4/1  "<slat>"
  Unary Minus/1 -> Vector Concatenate/1
